simulink model "MCU_Stateflow_Analog"  (R2022b)
settings: Solver=FixedStepDiscrete  StartTime=0.0  StopTime=inf  FixedStep=0.002  RelTol=1e-3
undefined symbols (not defined in the file): ANALOG, cAgeingMode, cCurrentLoopMode, cNoneMode, cParaRecogMode, cSingleBoardMode, cSpeedLoopMode, cTorqueLoopMode, cVvvfOpenMode, FAULT, POWER_ON, STANDBY, TESTBED, VEHICLE, WORKING
libraries: simulink x9, SignalEditorBlockLib x1
(part 3 of 4)

== stateflow chart MCU_Stateflow_Analog/测试/Task_2ms1/Process/McModeManage ==
  (default) -> (junction 10)
  (junction 267) -> (junction 270) [order 1] : [WorkCmdSource_ModeCmd==cTorqueLoopMode]
  (junction 265) -> (junction 267) : [CommandSource == VEHICLE]
  (junction 10) -> (junction 265) [order 2]
  (junction 10) -> (junction 12) [order 1] : [CommandSource == TESTBED]
  (junction 12) -> (junction 40) [order 1] : [WorkCmdSource_ModeCmd==cTorqueLoopMode]
  (junction 270) -> (junction 272) : {WorkStateMc_ModeSelect = cTorqueLoopMode;
      | WorkCmdMc_RunCmd = WorkCmdSource_RunCmd;
      | WorkCmdMc_TorqueCmd = WorkCmdSource_TorqueCmd;}
  (junction 267) -> (junction 274) [order 2] : {WorkStateMc_ModeSelect = cNoneMode;}
  (junction 10) -> (junction 289) [order 3] : [CommandSource == ANALOG]
  (junction 12) -> (junction 47) [order 2]
  (junction 40) -> (junction 43) : {WorkStateMc_ModeSelect = cTorqueLoopMode;
      | WorkCmdMc_RunCmd = WorkCmdSource_RunCmd;
      | WorkCmdMc_TorqueCmd = WorkCmdSource_TorqueCmd;}
  (junction 43) -> (junction 243)
  (junction 243) -> (junction 238)
  (junction 274) -> (junction 272)
  (junction 47) -> (junction 49) [order 1] : [WorkCmdSource_ModeCmd ==cSpeedLoopMode ]
  (junction 272) -> (junction 277) [order 2]
  (junction 272) -> (junction 277) [order 1] : [ZeroTorqueFlag == 1]
      | {WorkStateMc_ModeSelect = cTorqueLoopMode;
      | WorkCmdMc_RunCmd = WorkCmdSource_RunCmd;
      | WorkCmdMc_TorqueCmd = 0;}
  (junction 47) -> (junction 57) [order 2]
  (junction 49) -> (junction 54) : {WorkStateMc_ModeSelect = cSpeedLoopMode;
      | WorkCmdMc_RunCmd = WorkCmdSource_RunCmd;
      | WorkCmdMc_SpeedCmd = WorkCmdSource_SpeedCmd;}
  (junction 328) -> (junction 238) [order 1] : [WorkStateModeSelectBefore ~= cSpeedLoopMode]{SpeedCtrl_SpeedCmdFilter = SpeedCal_speed2ms}
  (junction 289) -> (junction 292)
  (junction 54) -> (junction 328)
  (junction 328) -> (junction 238) [order 2]
  (junction 238) -> (junction 233)
  (junction 292) -> (junction 296) [order 1] : [WorkCmdSource_ModeCmd == cTorqueLoopMode]
  (junction 277) -> (junction 322)
  (junction 292) -> (junction 302) [order 2]
  (junction 296) -> (junction 298) : {WorkStateMc_ModeSelect = cTorqueLoopMode;
      | WorkCmdMc_RunCmd = WorkCmdSource_RunCmd;
      | WorkCmdMc_TorqueCmd = WorkCmdSource_TorqueCmd;}
  (junction 57) -> (junction 59) [order 1] : [WorkCmdSource_ModeCmd ==cCurrentLoopMode ]
  (junction 57) -> (junction 78) [order 2]
  (junction 59) -> (junction 61) : {WorkStateMc_ModeSelect = cCurrentLoopMode;
      | WorkCmdMc_RunCmd = WorkCmdSource_RunCmd;}
  (junction 61) -> (junction 64) [order 1] : [CurrentPolarCoordinatesFlg ==1]
  (junction 298) -> (junction 300)
  (junction 61) -> (junction 71) [order 2] : {WorkCmdMc_IsdCmd = WorkCmdSource_IsdCmd;
      | WorkCmdMc_IsqCmd = WorkCmdSource_IsqCmd}
  (junction 64) -> (junction 66) : {WorkCmdMc_CurrentCmd = WorkCmdSource_CurrentCmd;
      | WorkCmdMc_ThetaCmd = WorkCmdSource_ThetaCmd;}
  (junction 300) -> (junction 308)
  (junction 302) -> (junction 304) [order 1] : [WorkCmdSource_ModeCmd == cSpeedLoopMode]
  (junction 66) -> (junction 71)
  (junction 302) -> (junction 311) [order 2]
  (junction 304) -> (junction 306) : {WorkStateMc_ModeSelect = cSpeedLoopMode;
      | WorkCmdMc_RunCmd = WorkCmdSource_RunCmd;
      | WorkCmdMc_TorqueCmd = WorkCmdSource_SpeedCmd;}
  (junction 71) -> (junction 74)
  (junction 74) -> (junction 233)
  (junction 233) -> (junction 228)
  (junction 306) -> (junction 308)
  (junction 308) -> (junction 313)
  (junction 78) -> (junction 81) [order 1] : [WorkCmdSource_ModeCmd ==cVvvfOpenMode ]
  (junction 78) -> (junction 87) [order 2]
  (junction 81) -> (junction 83) : {WorkStateMc_ModeSelect = cVvvfOpenMode;
      | WorkCmdMc_RunCmd = WorkCmdSource_RunCmd;
      | WorkCmdMc_FreqCmd = WorkCmdSource_FreqCmd;}
  (junction 313) -> (junction 311)
  (junction 311) -> (junction 317) [order 2]
  (junction 311) -> (junction 317) [order 1] : [ZeroTorqueFlag == 1]
      | {WorkStateMc_ModeSelect = cTorqueLoopMode;
      | WorkCmdMc_RunCmd = WorkCmdSource_RunCmd;
      | WorkCmdMc_TorqueCmd = 0;}
  (junction 83) -> (junction 228)
  (junction 228) -> (junction 223)
  (junction 317) -> (junction 319)
  (junction 87) -> (junction 89) [order 1] : [WorkCmdSource_ModeCmd ==cParaRecogMode ]
  (junction 87) -> (junction 94) [order 2]
  (junction 89) -> (junction 91) : {WorkStateMc_ModeSelect = cParaRecogMode;
      | WorkCmdMc_RunCmd = WorkCmdSource_RunCmd;}
  (junction 91) -> (junction 223)
  (junction 223) -> (junction 252)
  (junction 94) -> (junction 96) [order 1] : [WorkCmdSource_ModeCmd ==cSingleBoardMode ]
  (junction 94) -> (junction 100) [order 2]
  (junction 96) -> (junction 98) : {WorkStateMc_ModeSelect = cSingleBoardMode;
      | WorkCmdMc_RunCmd = WorkCmdSource_RunCmd;}
  (junction 98) -> (junction 252)
  (junction 252) -> (junction 254)
  (junction 100) -> (junction 102) [order 1] : [WorkCmdSource_ModeCmd ==cAgeingMode ]
  (junction 100) -> (junction 108) [order 2]
  (junction 102) -> (junction 104) : {WorkStateMc_ModeSelect = cAgeingMode;
      | WorkCmdMc_RunCmd = WorkCmdSource_RunCmd;
      | WorkCmdMc_CurrentCmd = WorkCmdSource_CurrentCmd;
      | WorkCmdMc_ThetaCmd = WorkCmdSource_ThetaCmd;
      | WorkCmdMc_FreqCmd = WorkCmdSource_FreqCmd;}
  (junction 104) -> (junction 254)
  (junction 254) -> (junction 256)
  (junction 108) -> (junction 110) [order 1] : [WorkCmdSource_ModeCmd ==cNoneMode ]
  (junction 108) -> (junction 262) [order 2] : {WorkStateMc_ModeSelect = cNoneMode;}
  (junction 110) -> (junction 112) : {WorkStateMc_ModeSelect = cAgeingMode;
      | WorkCmdMc_RunCmd = WorkCmdSource_RunCmd;}
  (junction 112) -> (junction 256)
  (junction 256) -> (junction 260)
  (junction 260) -> (junction 262)
  (junction 262) -> (junction 259)
  (junction 259) -> (junction 280) [order 2]
  (junction 259) -> (junction 280) [order 1] : [ZeroTorqueFlag == 1]
      | {WorkStateMc_ModeSelect = cTorqueLoopMode;
      | WorkCmdMc_RunCmd = WorkCmdSource_RunCmd;
      | WorkCmdMc_TorqueCmd = 0;}
  (junction 280) -> (junction 324)
  data: WorkCmdSource_ThetaCmd input; CommandSource input; WorkCmdSource_ModeCmd input; WorkCmdSource_RunCmd input; WorkCmdSource_TorqueCmd input; WorkCmdSource_CurrentCmd input; WorkCmdSource_FreqCmd input; WorkCmdSource_IsdCmd input; WorkCmdSource_IsqCmd input; WorkCmdSource_SpeedCmd input; TESTBED parameter; cTorqueLoopMode parameter; WorkStateMc_ModeSelect output =cNoneMode; cSpeedLoopMode parameter; WorkCmdMc_RunCmd output uint16; WorkCmdMc_TorqueCmd output single; WorkCmdMc_SpeedCmd output; cCurrentLoopMode parameter; WorkCmdMc_ThetaCmd output; WorkCmdMc_CurrentCmd output; CurrentPolarCoordinatesFlg input; WorkCmdMc_IsdCmd output; WorkCmdMc_IsqCmd output; cVvvfOpenMode parameter; WorkCmdMc_FreqCmd output; cParaRecogMode parameter; cAgeingMode parameter; cSingleBoardMode parameter; cNoneMode parameter; VEHICLE parameter; ZeroTorqueFlag input; SpeedCal_speed2ms input; ANALOG parameter; WorkStateModeSelectBefore input; SpeedCtrl_SpeedCmdFilter output

== stateflow chart MCU_Stateflow_Analog/测试/Task_2ms1/Process/WorkCmdJudge ==
  (default) -> (junction 1)
  (junction 10) -> (junction 31) [order 1] : [WorkState_TestBedWorkEn == 1]
  (junction 8) -> (junction 10) : [CommandSource ==TESTBED]
  (junction 1) -> (junction 8) [order 2]
  (junction 1) -> (junction 3) [order 1] : [CommandSource==VEHICLE]
  (junction 3) -> (junction 13) [order 1] : [WorkCmdVehicle_RunCmd == 1]
  (junction 31) -> (junction 34) : {WorkCmdSource_RunCmd =WorkCmdTestbed_RunCmd;
      | WorkCmdSource_DischargeCmd = WorkCmdTestbed_DischargeCmd;
      | WorkCmdSource_ModeCmd = WorkCmdTestbed_ModeCmd;
      | WorkCmdSource_TorqueCmd = WorkCmdTestbed_TorqueCmd;
      | WorkCmdSource_SpeedCmd = WorkCmdTestbed_SpeedCmd;
      | WorkCmdSource_CurrentCmd = WorkCmdTestbed_CurrentCmd;
      | WorkCmdSource_ThetaCmd = WorkCmdTestbed_ThetaCmd;
      | WorkCmdSource_IsdCmd = WorkCmdTestbed_IsdCmd;
      | WorkCmdSource_IsqCmd =WorkCmdTestbed_IsqCmd;
      | WorkCmdSource_FreqCmd = WorkCmdTestbed_FreqCmd;}
  (junction 10) -> (junction 36) [order 2] : {WorkCmdSource_RunCmd =0;
      | WorkCmdSource_DischargeCmd = 0;
      | WorkCmdSource_ModeCmd = cNoneMode;
      | WorkCmdSource_TorqueCmd = 0;
      | WorkCmdSource_SpeedCmd = 0;
      | WorkCmdSource_CurrentCmd = 0;
      | WorkCmdSource_ThetaCmd = 0;
      | WorkCmdSource_IsdCmd = 0;
      | WorkCmdSource_IsqCmd =0;
      | WorkCmdSource_FreqCmd = 0;}
  (junction 1) -> (junction 67) [order 3] : [CommandSource == ANALOG]
  (junction 3) -> (junction 28) [order 2] : {WorkCmdSource_RunCmd =0;
      | WorkCmdSource_DischargeCmd = WorkCmdVehicle_DischargeCmd;
      | WorkCmdSource_ModeCmd = cNoneMode;
      | WorkCmdSource_TorqueCmd = 0;
      | WorkCmdSource_SpeedCmd = 0;
      | WorkCmdSource_CurrentCmd = 0;
      | WorkCmdSource_ThetaCmd = 0;
      | WorkCmdSource_IsdCmd = 0;
      | WorkCmdSource_IsqCmd =0;
      | WorkCmdSource_FreqCmd = 0}
  (junction 13) -> (junction 15) : {WorkCmdSource_RunCmd =1;
      | WorkCmdSource_DischargeCmd = WorkCmdVehicle_DischargeCmd;
      | WorkCmdSource_ModeCmd = cTorqueLoopMode;
      | WorkCmdSource_TorqueCmd = WorkCmdVehicle_TorqueCmd
      | WorkCmdSource_SpeedCmd = 0;
      | WorkCmdSource_CurrentCmd = 0;
      | WorkCmdSource_ThetaCmd = 0;
      | WorkCmdSource_IsdCmd = 0;
      | WorkCmdSource_IsqCmd =0;
      | WorkCmdSource_FreqCmd = 0}
  (junction 36) -> (junction 34)
  (junction 28) -> (junction 15)
  (junction 34) -> (junction 56)
  (junction 15) -> (junction 54)
  (junction 67) -> (junction 70) [order 1] : [WorkCmdAnalog_RunCmd == 1]
  (junction 67) -> (junction 80) [order 2] : {WorkCmdSource_RunCmd =0;
      | WorkCmdSource_DischargeCmd = WorkCmdVehicle_DischargeCmd;
      | WorkCmdSource_ModeCmd = cNoneMode;
      | WorkCmdSource_TorqueCmd = 0;
      | WorkCmdSource_SpeedCmd = 0;
      | WorkCmdSource_CurrentCmd = 0;
      | WorkCmdSource_ThetaCmd = 0;
      | WorkCmdSource_IsdCmd = 0;
      | WorkCmdSource_IsqCmd =0;
      | WorkCmdSource_FreqCmd = 0}
  (junction 70) -> (junction 78) : {WorkCmdSource_RunCmd =1;
      | WorkCmdSource_DischargeCmd = 0;
      | WorkCmdSource_ModeCmd = WorkCmdAnalog_ModeCmd;
      | WorkCmdSource_TorqueCmd = WorkCmdAnalog_TorqueCmd;
      | WorkCmdSource_SpeedCmd = WorkCmdAnalog_SpeedCmd;
      | WorkCmdSource_CurrentCmd = 0;
      | WorkCmdSource_ThetaCmd = 0;
      | WorkCmdSource_IsdCmd = 0;
      | WorkCmdSource_IsqCmd =0;
      | WorkCmdSource_FreqCmd = 0}
  (junction 80) -> (junction 78)
  (junction 78) -> (junction 83)
  data: WorkCmdAnalog_ModeCmd input; CommandSource input int16; VEHICLE parameter int16; TESTBED parameter int16; WorkCmdVehicle_RunCmd input uint16; WorkCmdVehicle_DischargeCmd input uint16; WorkCmdSource_DischargeCmd output uint16; WorkCmdSource_RunCmd output uint16; WorkCmdSource_ModeCmd output uint16; cTorqueLoopMode parameter; WorkCmdSource_CurrentCmd output single; WorkCmdSource_FreqCmd output single; WorkCmdSource_IsdCmd output single; WorkCmdSource_IsqCmd output single; WorkCmdSource_SpeedCmd output single; WorkCmdSource_ThetaCmd output single; cNoneMode parameter; WorkState_TestBedWorkEn input uint16; WorkCmdTestbed_RunCmd input uint16; WorkCmdTestbed_DischargeCmd input uint16; WorkCmdTestbed_ModeCmd input uint16; WorkCmdTestbed_SpeedCmd input single; WorkCmdTestbed_CurrentCmd input single; WorkCmdTestbed_FreqCmd input single; WorkCmdTestbed_IsdCmd input single; WorkCmdTestbed_IsqCmd input single; WorkCmdTestbed_ThetaCmd input single; WorkCmdSource_TorqueCmd output single; WorkCmdVehicle_TorqueCmd input single; WorkCmdTestbed_TorqueCmd input single; WorkCmdAnalog_RunCmd input uint16; WorkCmdAnalog_SpeedCmd input; ANALOG parameter; WorkCmdAnalog_TorqueCmd input

== stateflow chart MCU_Stateflow_Analog/测试/Task_2ms1/草稿/Chart ==
  (default) -> (junction 10) : %差一个上一个周期的ModeSelect
      | {}
  (junction 10) -> (junction 12) : [CommandSource == TESTBED]
  (junction 12) -> (junction 40) [order 1] : [WorkCmdSource_ModeCmd==cTorqueLoopMode]
  (junction 12) -> (junction 47) [order 2]
  (junction 40) -> (junction 43) : {WorkStateMc_ModeSelect = cTorqueLoopMode;
      | WorkCmdMc_RunCmd = WorkCmdSource_RunCmd;
      | WorkCmdMc_TorqueCmd = WorkCmdSource_TorqueCmd;}
  (junction 43) -> (junction 243)
  (junction 243) -> (junction 245)
  (junction 47) -> (junction 49) [order 1] : [WorkCmdSource_ModeCmd ==cSpeedLoopMode ]
  (junction 47) -> (junction 57) [order 2]
  (junction 49) -> (junction 54) : {WorkStateMc_ModeSelect = cSpeedLoopMode;
      | WorkCmdMc_RunCmd = WorkCmdSource_RunCmd;
      | WorkCmdMc_SpeedCmd = WorkCmdSource_SpeedCmd;}
  (junction 54) -> (junction 238)
  (junction 238) -> (junction 240)
  (junction 57) -> (junction 59) [order 1] : [WorkCmdSource_ModeCmd ==cCurrentLoopMode ]
  (junction 57) -> (junction 78) [order 2]
  (junction 59) -> (junction 61) : {WorkStateMc_ModeSelect = cCurrentLoopMode;
      | WorkCmdMc_RunCmd = WorkCmdSource_RunCmd;}
  (junction 61) -> (junction 64) [order 1] : [CurrentPolarCoordinatesFlg ==1]
  (junction 61) -> (junction 71) [order 2] : {WorkCmdMc_IsdCmd = WorkCmdSource_IsdCmd;
      | WorkCmdMc_IsqCmd = WorkCmdSource_IsqCmd}
  (junction 64) -> (junction 66) : {WorkCmdMc_CurrentCmd = WorkCmdSource_CurrentCmd;
      | WorkCmdMc_ThetaCmd = WorkCmdSource_ThetaCmd;}
  (junction 66) -> (junction 71)
  (junction 71) -> (junction 74)
  (junction 74) -> (junction 233)
  (junction 233) -> (junction 235)
  (junction 78) -> (junction 81) [order 1] : [WorkCmdSource_ModeCmd ==cVvvfOpenMode ]
  (junction 78) -> (junction 87) [order 2]
  (junction 81) -> (junction 83) : {WorkStateMc_ModeSelect = cVvvfOpenMode;
      | WorkCmdMc_RunCmd = WorkCmdSource_RunCmd;
      | WorkCmdMc_FreqCmd = WorkCmdSource_FreqCmd;}
  (junction 83) -> (junction 228)
  (junction 228) -> (junction 230)
  (junction 87) -> (junction 89) [order 1] : [WorkCmdSource_ModeCmd ==cParaRecogMode ]
  (junction 87) -> (junction 94) [order 2]
  (junction 89) -> (junction 91) : {WorkStateMc_ModeSelect = cParaRecogMode;
      | WorkCmdMc_RunCmd = WorkCmdSource_RunCmd;}
  (junction 91) -> (junction 223)
  (junction 223) -> (junction 225)
  (junction 94) -> (junction 96) [order 1] : [WorkCmdSource_ModeCmd ==cSingleBoardMode ]
  (junction 94) -> (junction 100) [order 2]
  (junction 96) -> (junction 98) : {WorkStateMc_ModeSelect = cSingleBoardMode;
      | WorkCmdMc_RunCmd = WorkCmdSource_RunCmd;}
  (junction 98) -> (junction 218)
  (junction 218) -> (junction 220)
  (junction 100) -> (junction 102) [order 1] : [WorkCmdSource_ModeCmd ==cAgeingMode ]
  (junction 100) -> (junction 108) [order 2]
  (junction 102) -> (junction 104) : {WorkStateMc_ModeSelect = cAgeingMode;
      | WorkCmdMc_RunCmd = WorkCmdSource_RunCmd;
      | WorkCmdMc_CurrentCmd = WorkCmdSource_CurrentCmd;
      | WorkCmdMc_ThetaCmd = WorkCmdSource_ThetaCmd;
      | WorkCmdMc_FreqCmd = WorkCmdSource_FreqCmd;}
  (junction 104) -> (junction 213)
  (junction 213) -> (junction 215)
  (junction 108) -> (junction 110) [order 1] : [WorkCmdSource_ModeCmd ==cNoneMode ]
  (junction 108) -> (junction 114) [order 2] : {WorkStateMc_ModeSelect = cAgeingMode;}
  (junction 110) -> (junction 112) : {WorkStateMc_ModeSelect = cAgeingMode;
      | WorkCmdMc_RunCmd = WorkCmdSource_RunCmd;}
  (junction 112) -> (junction 114)
  (junction 215) -> (junction 112)
  (junction 220) -> (junction 215)
  (junction 225) -> (junction 220)
  (junction 230) -> (junction 225)
  (junction 235) -> (junction 230)
  (junction 240) -> (junction 235)
  (junction 245) -> (junction 240)
  (junction 114) -> (junction 211)
  data: WorkCmdSource_ThetaCmd input; CommandSource input; WorkCmdSource_ModeCmd input; WorkCmdSource_RunCmd input; WorkCmdSource_TorqueCmd input; WorkCmdSource_CurrentCmd input; WorkCmdSource_FreqCmd input; WorkCmdSource_IsdCmd input; WorkCmdSource_IsqCmd input; WorkCmdSource_SpeedCmd input; TESTBED parameter; cTorqueLoopMode parameter; WorkStateMc_ModeSelect output; cSpeedLoopMode parameter; WorkCmdMc_RunCmd output; WorkCmdMc_TorqueCmd output; WorkCmdMc_SpeedCmd output; cCurrentLoopMode parameter; WorkCmdMc_ThetaCmd output; WorkCmdMc_CurrentCmd output; CurrentPolarCoordinatesFlg input; WorkCmdMc_IsdCmd output; WorkCmdMc_IsqCmd output; cVvvfOpenMode parameter; WorkCmdMc_FreqCmd output; cParaRecogMode parameter; cAgeingMode parameter; cSingleBoardMode parameter; cNoneMode parameter

== stateflow chart MCU_Stateflow_Analog/测试/Task_2ms1/草稿/Chart2 ==
  (default) -> (junction 10) : %差一个上一个周期的ModeSelect
  (junction 10) -> (junction 12) [order 1] : [CommandSource == TESTBED]
  (junction 12) -> (junction 40) [order 1] : [WorkCmdSource_ModeCmd==cTorqueLoopMode]
  (junction 10) -> (junction 265) [order 2]
  (junction 12) -> (junction 47) [order 2]
  (junction 40) -> (junction 43) : {WorkStateMc_ModeSelect = cTorqueLoopMode;
      | WorkCmdMc_RunCmd = WorkCmdSource_RunCmd;
      | WorkCmdMc_TorqueCmd = WorkCmdSource_TorqueCmd;}
  (junction 43) -> (junction 243)
  (junction 267) -> (junction 270) [order 1] : [WorkCmdSource_ModeCmd==cTorqueLoopMode]
  (junction 265) -> (junction 267) : [CommandSource == VEHICLE]
  (junction 243) -> (junction 238)
  (junction 270) -> (junction 272) : {WorkStateMc_ModeSelect = cTorqueLoopMode;
      | WorkCmdMc_RunCmd = WorkCmdSource_RunCmd;
      | WorkCmdMc_TorqueCmd = WorkCmdSource_TorqueCmd;}
  (junction 267) -> (junction 274) [order 2] : {WorkStateMc_ModeSelect = cNoneMode;}
  (junction 47) -> (junction 49) [order 1] : [WorkCmdSource_ModeCmd ==cSpeedLoopMode ]
  (junction 47) -> (junction 57) [order 2]
  (junction 49) -> (junction 54) : {WorkStateMc_ModeSelect = cSpeedLoopMode;
      | WorkCmdMc_RunCmd = WorkCmdSource_RunCmd;
      | WorkCmdMc_SpeedCmd = WorkCmdSource_SpeedCmd;}
  (junction 274) -> (junction 272)
  (junction 54) -> (junction 238)
  (junction 272) -> (junction 277)
  (junction 238) -> (junction 233)
  (junction 57) -> (junction 59) [order 1] : [WorkCmdSource_ModeCmd ==cCurrentLoopMode ]
  (junction 57) -> (junction 78) [order 2]
  (junction 59) -> (junction 61) : {WorkStateMc_ModeSelect = cCurrentLoopMode;
      | WorkCmdMc_RunCmd = WorkCmdSource_RunCmd;}
  (junction 61) -> (junction 64) [order 1] : [CurrentPolarCoordinatesFlg ==1]
  (junction 61) -> (junction 71) [order 2] : {WorkCmdMc_IsdCmd = WorkCmdSource_IsdCmd;
      | WorkCmdMc_IsqCmd = WorkCmdSource_IsqCmd}
  (junction 64) -> (junction 66) : {WorkCmdMc_CurrentCmd = WorkCmdSource_CurrentCmd;
      | WorkCmdMc_ThetaCmd = WorkCmdSource_ThetaCmd;}
  (junction 66) -> (junction 71)
  (junction 71) -> (junction 74)
  (junction 74) -> (junction 233)
  (junction 233) -> (junction 228)
  (junction 78) -> (junction 81) [order 1] : [WorkCmdSource_ModeCmd ==cVvvfOpenMode ]
  (junction 78) -> (junction 87) [order 2]
  (junction 81) -> (junction 83) : {WorkStateMc_ModeSelect = cVvvfOpenMode;
      | WorkCmdMc_RunCmd = WorkCmdSource_RunCmd;
      | WorkCmdMc_FreqCmd = WorkCmdSource_FreqCmd;}
  (junction 83) -> (junction 228)
  (junction 228) -> (junction 223)
  (junction 87) -> (junction 89) [order 1] : [WorkCmdSource_ModeCmd ==cParaRecogMode ]
  (junction 87) -> (junction 94) [order 2]
  (junction 89) -> (junction 91) : {WorkStateMc_ModeSelect = cParaRecogMode;
      | WorkCmdMc_RunCmd = WorkCmdSource_RunCmd;}
  (junction 91) -> (junction 223)
  (junction 223) -> (junction 252)
  (junction 94) -> (junction 96) [order 1] : [WorkCmdSource_ModeCmd ==cSingleBoardMode ]
  (junction 94) -> (junction 100) [order 2]
  (junction 96) -> (junction 98) : {WorkStateMc_ModeSelect = cSingleBoardMode;
      | WorkCmdMc_RunCmd = WorkCmdSource_RunCmd;}
  (junction 98) -> (junction 252)
  (junction 252) -> (junction 254)
  (junction 100) -> (junction 102) [order 1] : [WorkCmdSource_ModeCmd ==cAgeingMode ]
  (junction 100) -> (junction 108) [order 2]
  (junction 102) -> (junction 104) : {WorkStateMc_ModeSelect = cAgeingMode;
      | WorkCmdMc_RunCmd = WorkCmdSource_RunCmd;
      | WorkCmdMc_CurrentCmd = WorkCmdSource_CurrentCmd;
      | WorkCmdMc_ThetaCmd = WorkCmdSource_ThetaCmd;
      | WorkCmdMc_FreqCmd = WorkCmdSource_FreqCmd;}
  (junction 104) -> (junction 254)
  (junction 254) -> (junction 256)
  (junction 108) -> (junction 110) [order 1] : [WorkCmdSource_ModeCmd ==cNoneMode ]
  (junction 108) -> (junction 262) [order 2] : {WorkStateMc_ModeSelect = cNoneMode;}
  (junction 110) -> (junction 112) : {WorkStateMc_ModeSelect = cAgeingMode;
      | WorkCmdMc_RunCmd = WorkCmdSource_RunCmd;}
  (junction 112) -> (junction 256)
  (junction 256) -> (junction 260)
  (junction 260) -> (junction 262)
  (junction 262) -> (junction 259)
  data: WorkCmdSource_ThetaCmd input; CommandSource input; WorkCmdSource_ModeCmd input; WorkCmdSource_RunCmd input; WorkCmdSource_TorqueCmd input; WorkCmdSource_CurrentCmd input; WorkCmdSource_FreqCmd input; WorkCmdSource_IsdCmd input; WorkCmdSource_IsqCmd input; WorkCmdSource_SpeedCmd input; TESTBED parameter; cTorqueLoopMode parameter; WorkStateMc_ModeSelect output; cSpeedLoopMode parameter; WorkCmdMc_RunCmd output; WorkCmdMc_TorqueCmd output; WorkCmdMc_SpeedCmd output; cCurrentLoopMode parameter; WorkCmdMc_ThetaCmd output; WorkCmdMc_CurrentCmd output; CurrentPolarCoordinatesFlg input; WorkCmdMc_IsdCmd output; WorkCmdMc_IsqCmd output; cVvvfOpenMode parameter; WorkCmdMc_FreqCmd output; cParaRecogMode parameter; cAgeingMode parameter; cSingleBoardMode parameter; cNoneMode parameter; VEHICLE parameter

== stateflow chart MCU_Stateflow_Analog/测试/Task_2ms1/草稿/MotorState1 ==
  state PowerOn
    WorkState_WorkState = POWER_ON
  state Fault
    WorkState_WorkState = FAULT;
  state StandBy
    WorkState_WorkState = STANDBY;
  state Working
    WorkState_WorkState = WORKING;
  (default) -> PowerOn
  PowerOn -> (junction 21) : [SelfCheck_OverFlg == 1]
  (junction 13) -> Fault : {WorkState_WorkState = FAULT;
      | WorkState_WorkStateBefore = POWER_ON;
      | WorkState_ModeSelect = cNoneMode;}
  (junction 21) -> (junction 13) [order 1] : [ClosePWMFlag == 1]
  (junction 21) -> StandBy [order 2] : {WorkState_WorkState = STANDBY;
      | WorkState_WorkStateBefore = POWER_ON;
      | WorkState_ModeSelect = cNoneMode;}
  (junction 26) -> Fault : {WorkState_WorkState = FAULT;
      | WorkState_WorkStateBefore = STANDBY;
      | WorkState_ModeSelect = cNoneMode}
  StandBy -> (junction 26) [order 1] : [ClosePWMFlag ==1]
  Fault -> (junction 47) : [ClosePWMFlag ==0]
  (junction 47) -> StandBy : {WorkState_WorkState = STANDBY;
      | WorkState_WorkStateBefore = FAULT;
      | WorkState_ModeSelect = cNoneMode}
  StandBy -> (junction 30) [order 2] : [(WorkCmdSource_ModeCmd ~=cNoneMode & WorkCmdSource_RunCmd==true &Precharge_PrechargeOver==true) ||(WormCmdSource_ModeCmd ==cSingleBoardMode)]
  (junction 30) -> Working : {WorkState_WorkState =WORKING;
      | WorkState_WorkStateBefore = STANDBY;}
  (junction 43) -> Fault : {WorkState_WorkState = FAULT;
      | WorkState_WorkStateBefore = WORKING;
      | WorkState_ModeSelect = cNoneMode;}
  Working -> (junction 43) : [ClosePWMFlag==1]
  data: SelfCheck_OverFlg input; POWER_ON parameter; ClosePWMFlag input; FAULT parameter; WorkState_WorkState output; WorkState_WorkStateBefore output; cNoneMode parameter; WorkState_ModeSelect output; STANDBY parameter; cSingleBoardMode parameter; WormCmdSource_ModeCmd input; WorkCmdSource_RunCmd input; WorkCmdSource_ModeCmd input; Precharge_PrechargeOver input; WORKING parameter

== stateflow chart MCU_Stateflow_Analog/测试/Task_2ms1/草稿/MotorState2 ==
  state PowerOn
    WorkState_WorkState = POWER_ON
  state Fault
    WorkState_WorkState = FAULT;
  state StandBy
    WorkState_WorkState = STANDBY;
  state Working
    WorkState_WorkState = WORKING;
  (default) -> PowerOn
  PowerOn -> (junction 21) : [SelfCheck_OverFlg == 1]
  (junction 13) -> Fault : {WorkState_WorkState = FAULT;
      | WorkState_WorkStateBefore = POWER_ON;
      | WorkState_ModeSelect = cNoneMode;}
  (junction 21) -> (junction 13) [order 1] : [ClosePWMFlag == 1]
  (junction 21) -> StandBy [order 2] : {WorkState_WorkState = STANDBY;
      | WorkState_WorkStateBefore = POWER_ON;
      | WorkState_ModeSelect = cNoneMode;}
  (junction 26) -> Fault : {WorkState_WorkState = FAULT;
      | WorkState_WorkStateBefore = STANDBY;
      | WorkState_ModeSelect = cNoneMode}
  StandBy -> (junction 26) [order 1] : [ClosePWMFlag ==1]
  Fault -> (junction 47) : [ClosePWMFlag ==0]
  (junction 47) -> StandBy : {WorkState_WorkState = STANDBY;
      | WorkState_WorkStateBefore = FAULT;
      | WorkState_ModeSelect = cNoneMode}
  StandBy -> (junction 30) [order 2] : [(WorkCmdSource_ModeCmd ~=cNoneMode & WorkCmdSource_RunCmd==true &Precharge_PrechargeOver==true) ||(WormCmdSource_ModeCmd ==cSingleBoardMode)]
  (junction 30) -> Working : {WorkState_WorkState =WORKING;
      | WorkState_WorkStateBefore = STANDBY;}
  (junction 43) -> Fault : {WorkState_WorkState = FAULT;
      | WorkState_WorkStateBefore = WORKING;
      | WorkState_ModeSelect = cNoneMode;}
  Working -> (junction 43) : [ClosePWMFlag==1]
  data: WorkCmdMc_FreqCmd input; WorkCmdMc_IsqCmd input; WorkCmdMc_IsdCmd input; WorkCmdMc_CurrentCmd input; WorkCmdMc_ThetaCmd input; WorkCmdMc_TorqueCmd input; SelfCheck_OverFlg input; POWER_ON parameter; ClosePWMFlag input; FAULT parameter; WorkState_WorkState output; WorkState_WorkStateBefore output; cNoneMode parameter; WorkState_ModeSelect output; STANDBY parameter; cSingleBoardMode parameter; WormCmdSource_ModeCmd input; WorkCmdSource_RunCmd input; WorkCmdSource_ModeCmd input; Precharge_PrechargeOver input; WORKING parameter; WorkStateMc_ModeSelect input; WorkCmdMc_RunCmd input; WorkCmdMc_SpeedCmd input

== stateflow chart MCU_Stateflow_Analog/测试/Task_2ms1/草稿/MotorState3 ==
  state PowerOn
    WorkState_WorkState = POWER_ON
    %WorkCmd_RunCmd = WorkCmdMc_RunCmd;
    %WorkCmd_DischargeCmd = 0;
    %WorkCmd_ModeCmd = cNoneMode;
    %WorkCmd_TorqueCmd = 0;
    %WorkCmd_SpeedCmd = 0;
    %WorkCmd_CurrentCmd = 0;
    %WorkCmd_ThetaCmd = 0;
    %WorkCmd_IsdCmd = 0;
    %WorkCmd_IsqCmd = 0;
    %WorkCmd_FreqCmd = 0;
  state Fault
    %WorkState_WorkState = FAULT;
    %WorkState_WorkState = FAULT;
    %WorkCmd_RunCmd = WorkCmdMc_RunCmd;
    %WorkCmd_DischargeCmd = 0;
    %WorkCmd_ModeCmd = cNoneMode;
    %WorkCmd_TorqueCmd = 0;
    %WorkCmd_SpeedCmd = 0;
    %WorkCmd_CurrentCmd = 0;
    %WorkCmd_ThetaCmd = 0;
    %WorkCmd_IsdCmd = 0;
    %WorkCmd_IsqCmd = 0;
    %WorkCmd_FreqCmd = 0;
  state StandBy
    WorkState_WorkState = STANDBY;
  state Working
    WorkState_WorkState = WORKING;
  (default) -> PowerOn
  PowerOn -> (junction 21) : [SelfCheck_OverFlg == 1]
  (junction 13) -> Fault : {WorkState_WorkState = FAULT;
      | WorkState_WorkStateBefore = POWER_ON;
      | WorkState_ModeSelect = cNoneMode;}
  (junction 21) -> (junction 13) [order 1] : [ClosePWMFlag == 1]
  (junction 21) -> StandBy [order 2] : {WorkState_WorkState = STANDBY;
      | WorkState_WorkStateBefore = POWER_ON;
      | WorkState_ModeSelect = cNoneMode;}
  StandBy -> (junction 26) [order 1] : [ClosePWMFlag ==1]
  (junction 26) -> Fault : {WorkState_WorkState = FAULT;
      | WorkState_WorkStateBefore = STANDBY;
      | WorkState_ModeSelect = cNoneMode}
  Fault -> (junction 47) : [ClosePWMFlag ==0]
  (junction 47) -> StandBy : {WorkState_WorkState = STANDBY;
      | WorkState_WorkStateBefore = FAULT;
      | WorkState_ModeSelect = cNoneMode}
  StandBy -> (junction 30) [order 2] : [(WorkCmdSource_ModeCmd ~=cNoneMode & WorkCmdSource_RunCmd==true &Precharge_PrechargeOver==true) ||(WorkCmdSource_ModeCmd ==cSingleBoardMode)]
  (junction 72) -> StandBy : {WorkState_WorkState = STANDBY;
      | WorkState_WorkStateBefore = WORKING;
      | WorkState_ModeSelect = cNoneMode;}
  (junction 30) -> Working : {WorkState_WorkState =WORKING;
      | WorkState_WorkStateBefore = STANDBY;}
  Working -> (junction 72) [order 2] : [(WorkCmdSource_RunCmd ==false & WorkState_ModeSelect ~= cSingleBoardMode) || (WorkState_ModeSelect == cNoneMode)]
  (junction 43) -> Fault : {WorkState_WorkState = FAULT;
      | WorkState_WorkStateBefore = WORKING;
      | WorkState_ModeSelect = cNoneMode;}
  Working -> (junction 43) [order 1] : [ClosePWMFlag==1]
  data: SelfCheck_OverFlg input; POWER_ON parameter; ClosePWMFlag input; FAULT parameter; WorkState_WorkState output; WorkState_WorkStateBefore output; cNoneMode parameter; WorkState_ModeSelect output; STANDBY parameter; cSingleBoardMode parameter; WorkCmdSource_RunCmd input; WorkCmdSource_ModeCmd input; Precharge_PrechargeOver input; WORKING parameter

== stateflow chart MCU_Stateflow_Analog/测试/Task_2ms1/草稿/MotorState4 ==
  state PowerOn
    %包括Sensor_Self_Check和Ctrl_Reset
    WorkState_WorkState = POWER_ON
  state Fault
    %WorkState_WorkState = FAULT;
    %{
    WorkState_WorkState = FAULT;
    WorkCmd_RunCmd = WorkCmdMc_RunCmd;
    WorkCmd_DischargeCmd = 0;
    WorkCmd_ModeCmd = cNoneMode;
    WorkCmd_TorqueCmd = 0;
    WorkCmd_SpeedCmd = 0;
    WorkCmd_CurrentCmd = 0;
    WorkCmd_ThetaCmd = 0;
    WorkCmd_IsdCmd = 0;
    WorkCmd_IsqCmd = 0;
    WorkCmd_FreqCmd = 0;
    %}
  state StandBy
    WorkState_WorkState = STANDBY;
  state Working
    WorkState_WorkState = WORKING;
  (default) -> PowerOn
  PowerOn -> (junction 21) : [SelfCheck_OverFlg == 1]
  (junction 13) -> Fault : {WorkState_WorkState = FAULT;
      | WorkState_WorkStateBefore = POWER_ON;
      | WorkState_ModeSelect = cNoneMode;}
  (junction 21) -> (junction 13) [order 1] : [ClosePWMFlag == 1]
  (junction 21) -> StandBy [order 2] : {
      | WorkState_WorkState = STANDBY;
      | WorkState_WorkStateBefore = POWER_ON;
      | WorkState_ModeSelect = cNoneMode;}
  StandBy -> (junction 26) [order 1] : [ClosePWMFlag ==1]
  (junction 26) -> Fault : {WorkState_WorkState = FAULT;
      | WorkState_WorkStateBefore = STANDBY;
      | WorkState_ModeSelect = cNoneMode}
  Fault -> (junction 47) : [ClosePWMFlag ==0]
  (junction 47) -> StandBy : {WorkState_WorkState = STANDBY;
      | WorkState_WorkStateBefore = FAULT;
      | WorkState_ModeSelect = cNoneMode}
  StandBy -> (junction 30) [order 2] : [(WorkCmdSource_ModeCmd ~=cNoneMode & WorkCmdSource_RunCmd==true &Precharge_PrechargeOver==true) ||(WorkCmdSource_ModeCmd ==cSingleBoardMode)]
  (junction 72) -> StandBy : {WorkState_WorkState = STANDBY;
      | WorkState_WorkStateBefore = POWER_ON;
      | WorkState_ModeSelect = cNoneMode;}
  (junction 30) -> Working : {WorkState_WorkState =WORKING;
      | WorkState_WorkStateBefore = STANDBY;}
  Working -> (junction 72) [order 2] : [(WorkCmdSource_RunCmd ==false & WorkState_ModeSelect ~= cSingleBoardMode) || (WorkState_ModeSelect == cNoneMode)]
  (junction 43) -> Fault : {WorkState_WorkState = FAULT;
      | WorkState_WorkStateBefore = WORKING;
      | WorkState_ModeSelect = cNoneMode;}
  Working -> (junction 43) [order 1] : [ClosePWMFlag==1]
  data: SelfCheck_OverFlg input; POWER_ON parameter; ClosePWMFlag input; FAULT parameter; WorkState_WorkState output; WorkState_WorkStateBefore output; cNoneMode parameter; WorkState_ModeSelect output; STANDBY parameter; cSingleBoardMode parameter; WorkCmdSource_RunCmd input; WorkCmdSource_ModeCmd input; Precharge_PrechargeOver input; WORKING parameter

== stateflow chart MCU_Stateflow_Analog/测试/Task_2ms2/MotorState ==
  state PowerOn
    %包括Sensor_Self_Check和Ctrl_Reset
    WorkState_WorkState = POWER_ON;
  state Fault
    %WorkState_WorkState = FAULT;
    %{
    WorkState_WorkState = FAULT;
    WorkCmd_RunCmd = WorkCmdMc_RunCmd;
    WorkCmd_DischargeCmd = 0;
    WorkCmd_ModeCmd = cNoneMode;
    WorkCmd_TorqueCmd = 0;
    WorkCmd_SpeedCmd = 0;
    WorkCmd_CurrentCmd = 0;
    WorkCmd_ThetaCmd = 0;
    WorkCmd_IsdCmd = 0;
    WorkCmd_IsqCmd = 0;
    WorkCmd_FreqCmd = 0;
    %}
  state StandBy
    WorkState_WorkState = STANDBY;
  state Working
    WorkState_WorkState = WORKING;
  (default) -> PowerOn
  PowerOn -> (junction 21) : [SelfCheck_OverFlg == 1]
  (junction 13) -> Fault : {
      | WorkState_WorkState = FAULT;
      | WorkState_WorkStateBefore = POWER_ON;
      | %WorkState_ModeSelect = cNoneMode;
      | }
  (junction 21) -> (junction 13) [order 1] : [ClosePWMFlag == 1]
  (junction 21) -> StandBy [order 2] : {
      | WorkState_WorkState = STANDBY;
      | WorkState_WorkStateBefore = POWER_ON;
      | %WorkState_ModeSelect = cNoneMode;
      | }
  StandBy -> (junction 26) [order 1] : [ClosePWMFlag ==1]
  (junction 26) -> Fault : {
      | WorkState_WorkState = FAULT;
      | WorkState_WorkStateBefore = STANDBY;
      | %WorkState_ModeSelect = cNoneMode
      | }
  Fault -> (junction 47) : [ClosePWMFlag ==0]
  (junction 47) -> StandBy : {
      | WorkState_WorkState = STANDBY;
      | WorkState_WorkStateBefore = FAULT;
      | %WorkState_ModeSelect = cNoneMode
      | }
  StandBy -> (junction 30) [order 2] : [(WorkCmdSource_ModeCmd ~=cNoneMode & WorkCmdSource_RunCmd==true &Precharge_PrechargeOver==true) ||(WorkCmdSource_ModeCmd ==cSingleBoardMode)]
  (junction 72) -> StandBy : {
      | WorkState_WorkState = STANDBY;
      | WorkState_WorkStateBefore = POWER_ON;
      | %WorkState_ModeSelect = cNoneMode;
      | }
  (junction 30) -> Working : {WorkState_WorkState =WORKING;
      | WorkState_WorkStateBefore = STANDBY;}
  Working -> (junction 72) [order 2] : %[(WorkCmdSource_RunCmd ==false & WorkState_ModeSelect ~= cSingleBoardMode) || (WorkState_ModeSelect == cNoneMode)]
      | [(WorkCmdSource_RunCmd ==false & WorkStateMc_ModeSelect ~= cSingleBoardMode) || (WorkStateMc_ModeSelect == cNoneMode)]
  (junction 43) -> Fault : {WorkState_WorkState = FAULT;
      | WorkState_WorkStateBefore = WORKING;
      | %WorkState_ModeSelect = cNoneMode;
      | }
  Working -> (junction 43) [order 1] : [ClosePWMFlag==1]
  data: SelfCheck_OverFlg input; POWER_ON parameter; ClosePWMFlag input; FAULT parameter; WorkState_WorkState output; WorkState_WorkStateBefore output; cNoneMode parameter; STANDBY parameter; cSingleBoardMode parameter; WorkCmdSource_RunCmd input; WorkCmdSource_ModeCmd input; Precharge_PrechargeOver input; WORKING parameter; WorkStateMc_ModeSelect input

== stateflow chart MCU_Stateflow_Analog/测试/Task_2ms2/Process/McModeManage ==
  (default) -> (junction 10)
  (junction 267) -> (junction 270) [order 1] : [WorkCmdSource_ModeCmd==cTorqueLoopMode]
  (junction 265) -> (junction 267) : [CommandSource == VEHICLE]
  (junction 10) -> (junction 265) [order 2]
  (junction 10) -> (junction 12) [order 1] : [CommandSource == TESTBED]
  (junction 12) -> (junction 40) [order 1] : [WorkCmdSource_ModeCmd==cTorqueLoopMode]
  (junction 270) -> (junction 272) : {WorkStateMc_ModeSelect = cTorqueLoopMode;
      | WorkCmdMc_RunCmd = WorkCmdSource_RunCmd;
      | WorkCmdMc_TorqueCmd = WorkCmdSource_TorqueCmd;}
  (junction 267) -> (junction 274) [order 2] : {WorkStateMc_ModeSelect = cNoneMode;}
  (junction 10) -> (junction 289) [order 3] : [CommandSource == ANALOG]
  (junction 12) -> (junction 47) [order 2]
  (junction 40) -> (junction 43) : {WorkStateMc_ModeSelect = cTorqueLoopMode;
      | WorkCmdMc_RunCmd = WorkCmdSource_RunCmd;
      | WorkCmdMc_TorqueCmd = WorkCmdSource_TorqueCmd;}
  (junction 43) -> (junction 243)
  (junction 243) -> (junction 238)
  (junction 274) -> (junction 272)
  (junction 47) -> (junction 49) [order 1] : [WorkCmdSource_ModeCmd ==cSpeedLoopMode ]
  (junction 272) -> (junction 277) [order 2]
  (junction 272) -> (junction 277) [order 1] : [ZeroTorqueFlag == 1]
      | {WorkStateMc_ModeSelect = cTorqueLoopMode;
      | WorkCmdMc_RunCmd = WorkCmdSource_RunCmd;
      | WorkCmdMc_TorqueCmd = 0;}
  (junction 47) -> (junction 57) [order 2]
  (junction 49) -> (junction 54) : {WorkStateMc_ModeSelect = cSpeedLoopMode;
      | WorkCmdMc_RunCmd = WorkCmdSource_RunCmd;
      | WorkCmdMc_SpeedCmd = WorkCmdSource_SpeedCmd;}
  (junction 328) -> (junction 238) [order 1] : [WorkStateModeSelectBefore ~= cSpeedLoopMode]{SpeedCtrl_SpeedCmdFilter = SpeedCal_speed2ms}
  (junction 289) -> (junction 292)
  (junction 54) -> (junction 328)
  (junction 328) -> (junction 238) [order 2]
  (junction 238) -> (junction 233)
  (junction 292) -> (junction 296) [order 1] : [WorkCmdSource_ModeCmd == cTorqueLoopMode]
  (junction 277) -> (junction 322)
  (junction 292) -> (junction 302) [order 2]
  (junction 296) -> (junction 298) : {WorkStateMc_ModeSelect = cTorqueLoopMode;
      | WorkCmdMc_RunCmd = WorkCmdSource_RunCmd;
      | WorkCmdMc_TorqueCmd = WorkCmdSource_TorqueCmd;}
  (junction 57) -> (junction 59) [order 1] : [WorkCmdSource_ModeCmd ==cCurrentLoopMode ]
  (junction 57) -> (junction 78) [order 2]
  (junction 59) -> (junction 61) : {WorkStateMc_ModeSelect = cCurrentLoopMode;
      | WorkCmdMc_RunCmd = WorkCmdSource_RunCmd;}
  (junction 61) -> (junction 64) [order 1] : [CurrentPolarCoordinatesFlg ==1]
  (junction 298) -> (junction 300)
  (junction 61) -> (junction 71) [order 2] : {WorkCmdMc_IsdCmd = WorkCmdSource_IsdCmd;
      | WorkCmdMc_IsqCmd = WorkCmdSource_IsqCmd}
  (junction 64) -> (junction 66) : {WorkCmdMc_CurrentCmd = WorkCmdSource_CurrentCmd;
      | WorkCmdMc_ThetaCmd = WorkCmdSource_ThetaCmd;}
  (junction 300) -> (junction 308)
  (junction 302) -> (junction 304) [order 1] : [WorkCmdSource_ModeCmd == cSpeedLoopMode]
  (junction 66) -> (junction 71)
  (junction 302) -> (junction 311) [order 2]
  (junction 304) -> (junction 306) : {WorkStateMc_ModeSelect = cSpeedLoopMode;
      | WorkCmdMc_RunCmd = WorkCmdSource_RunCmd;
      | WorkCmdMc_TorqueCmd = WorkCmdSource_SpeedCmd;}
  (junction 71) -> (junction 74)
  (junction 74) -> (junction 233)
  (junction 233) -> (junction 228)
  (junction 306) -> (junction 308)
  (junction 308) -> (junction 313)
  (junction 78) -> (junction 81) [order 1] : [WorkCmdSource_ModeCmd ==cVvvfOpenMode ]
  (junction 78) -> (junction 87) [order 2]
  (junction 81) -> (junction 83) : {WorkStateMc_ModeSelect = cVvvfOpenMode;
      | WorkCmdMc_RunCmd = WorkCmdSource_RunCmd;
      | WorkCmdMc_FreqCmd = WorkCmdSource_FreqCmd;}
  (junction 313) -> (junction 311)
  (junction 311) -> (junction 317) [order 2]
  (junction 311) -> (junction 317) [order 1] : [ZeroTorqueFlag == 1]
      | {WorkStateMc_ModeSelect = cTorqueLoopMode;
      | WorkCmdMc_RunCmd = WorkCmdSource_RunCmd;
      | WorkCmdMc_TorqueCmd = 0;}
  (junction 83) -> (junction 228)
  (junction 228) -> (junction 223)
  (junction 317) -> (junction 319)
  (junction 87) -> (junction 89) [order 1] : [WorkCmdSource_ModeCmd ==cParaRecogMode ]
  (junction 87) -> (junction 94) [order 2]
  (junction 89) -> (junction 91) : {WorkStateMc_ModeSelect = cParaRecogMode;
      | WorkCmdMc_RunCmd = WorkCmdSource_RunCmd;}
  (junction 91) -> (junction 223)
  (junction 223) -> (junction 252)
  (junction 94) -> (junction 96) [order 1] : [WorkCmdSource_ModeCmd ==cSingleBoardMode ]
  (junction 94) -> (junction 100) [order 2]
  (junction 96) -> (junction 98) : {WorkStateMc_ModeSelect = cSingleBoardMode;
      | WorkCmdMc_RunCmd = WorkCmdSource_RunCmd;}
  (junction 98) -> (junction 252)
  (junction 252) -> (junction 254)
  (junction 100) -> (junction 102) [order 1] : [WorkCmdSource_ModeCmd ==cAgeingMode ]
  (junction 100) -> (junction 108) [order 2]
  (junction 102) -> (junction 104) : {WorkStateMc_ModeSelect = cAgeingMode;
      | WorkCmdMc_RunCmd = WorkCmdSource_RunCmd;
      | WorkCmdMc_CurrentCmd = WorkCmdSource_CurrentCmd;
      | WorkCmdMc_ThetaCmd = WorkCmdSource_ThetaCmd;
      | WorkCmdMc_FreqCmd = WorkCmdSource_FreqCmd;}
  (junction 104) -> (junction 254)
  (junction 254) -> (junction 256)
  (junction 108) -> (junction 110) [order 1] : [WorkCmdSource_ModeCmd ==cNoneMode ]
  (junction 108) -> (junction 262) [order 2] : {WorkStateMc_ModeSelect = cNoneMode;}
  (junction 110) -> (junction 112) : {WorkStateMc_ModeSelect = cAgeingMode;
      | WorkCmdMc_RunCmd = WorkCmdSource_RunCmd;}
  (junction 112) -> (junction 256)
  (junction 256) -> (junction 260)
  (junction 260) -> (junction 262)
  (junction 262) -> (junction 259)
  (junction 259) -> (junction 280) [order 2]
  (junction 259) -> (junction 280) [order 1] : [ZeroTorqueFlag == 1]
      | {WorkStateMc_ModeSelect = cTorqueLoopMode;
      | WorkCmdMc_RunCmd = WorkCmdSource_RunCmd;
      | WorkCmdMc_TorqueCmd = 0;}
  (junction 280) -> (junction 324)
  data: WorkCmdSource_ThetaCmd input; CommandSource input; WorkCmdSource_ModeCmd input; WorkCmdSource_RunCmd input; WorkCmdSource_TorqueCmd input; WorkCmdSource_CurrentCmd input; WorkCmdSource_FreqCmd input; WorkCmdSource_IsdCmd input; WorkCmdSource_IsqCmd input; WorkCmdSource_SpeedCmd input; TESTBED parameter; cTorqueLoopMode parameter; WorkStateMc_ModeSelect output =cNoneMode; cSpeedLoopMode parameter; WorkCmdMc_RunCmd output uint16; WorkCmdMc_TorqueCmd output single; WorkCmdMc_SpeedCmd output; cCurrentLoopMode parameter; WorkCmdMc_ThetaCmd output; WorkCmdMc_CurrentCmd output; CurrentPolarCoordinatesFlg input; WorkCmdMc_IsdCmd output; WorkCmdMc_IsqCmd output; cVvvfOpenMode parameter; WorkCmdMc_FreqCmd output; cParaRecogMode parameter; cAgeingMode parameter; cSingleBoardMode parameter; cNoneMode parameter; VEHICLE parameter; ZeroTorqueFlag input; SpeedCal_speed2ms input; ANALOG parameter; WorkStateModeSelectBefore input; SpeedCtrl_SpeedCmdFilter output

== stateflow chart MCU_Stateflow_Analog/测试/Task_2ms2/Process/WorkCmdJudge ==
  (default) -> (junction 1)
  (junction 10) -> (junction 31) [order 1] : [WorkState_TestBedWorkEn == 1]
  (junction 8) -> (junction 10) : [CommandSource ==TESTBED]
  (junction 1) -> (junction 8) [order 2]
  (junction 1) -> (junction 3) [order 1] : [CommandSource==VEHICLE]
  (junction 3) -> (junction 13) [order 1] : [WorkCmdVehicle_RunCmd == 1]
  (junction 31) -> (junction 34) : {WorkCmdSource_RunCmd =WorkCmdTestbed_RunCmd;
      | WorkCmdSource_DischargeCmd = WorkCmdTestbed_DischargeCmd;
      | WorkCmdSource_ModeCmd = WorkCmdTestbed_ModeCmd;
      | WorkCmdSource_TorqueCmd = WorkCmdTestbed_TorqueCmd;
      | WorkCmdSource_SpeedCmd = WorkCmdTestbed_SpeedCmd;
      | WorkCmdSource_CurrentCmd = WorkCmdTestbed_CurrentCmd;
      | WorkCmdSource_ThetaCmd = WorkCmdTestbed_ThetaCmd;
      | WorkCmdSource_IsdCmd = WorkCmdTestbed_IsdCmd;
      | WorkCmdSource_IsqCmd =WorkCmdTestbed_IsqCmd;
      | WorkCmdSource_FreqCmd = WorkCmdTestbed_FreqCmd;}
  (junction 10) -> (junction 36) [order 2] : {WorkCmdSource_RunCmd =0;
      | WorkCmdSource_DischargeCmd = 0;
      | WorkCmdSource_ModeCmd = cNoneMode;
      | WorkCmdSource_TorqueCmd = 0;
      | WorkCmdSource_SpeedCmd = 0;
      | WorkCmdSource_CurrentCmd = 0;
      | WorkCmdSource_ThetaCmd = 0;
      | WorkCmdSource_IsdCmd = 0;
      | WorkCmdSource_IsqCmd =0;
      | WorkCmdSource_FreqCmd = 0;}
  (junction 1) -> (junction 67) [order 3] : [CommandSource == ANALOG]
  (junction 3) -> (junction 28) [order 2] : {WorkCmdSource_RunCmd =0;
      | WorkCmdSource_DischargeCmd = WorkCmdVehicle_DischargeCmd;
      | WorkCmdSource_ModeCmd = cNoneMode;
      | WorkCmdSource_TorqueCmd = 0;
      | WorkCmdSource_SpeedCmd = 0;
      | WorkCmdSource_CurrentCmd = 0;
      | WorkCmdSource_ThetaCmd = 0;
      | WorkCmdSource_IsdCmd = 0;
      | WorkCmdSource_IsqCmd =0;
      | WorkCmdSource_FreqCmd = 0}
  (junction 13) -> (junction 15) : {WorkCmdSource_RunCmd =1;
      | WorkCmdSource_DischargeCmd = WorkCmdVehicle_DischargeCmd;
      | WorkCmdSource_ModeCmd = cTorqueLoopMode;
      | WorkCmdSource_TorqueCmd = WorkCmdVehicle_TorqueCmd
      | WorkCmdSource_SpeedCmd = 0;
      | WorkCmdSource_CurrentCmd = 0;
      | WorkCmdSource_ThetaCmd = 0;
      | WorkCmdSource_IsdCmd = 0;
      | WorkCmdSource_IsqCmd =0;
      | WorkCmdSource_FreqCmd = 0}
  (junction 36) -> (junction 34)
  (junction 28) -> (junction 15)
  (junction 34) -> (junction 56)
  (junction 15) -> (junction 54)
  (junction 67) -> (junction 70) [order 1] : [WorkCmdAnalog_RunCmd == 1]
  (junction 67) -> (junction 80) [order 2] : {WorkCmdSource_RunCmd =0;
      | WorkCmdSource_DischargeCmd = WorkCmdVehicle_DischargeCmd;
      | WorkCmdSource_ModeCmd = cNoneMode;
      | WorkCmdSource_TorqueCmd = 0;
      | WorkCmdSource_SpeedCmd = 0;
      | WorkCmdSource_CurrentCmd = 0;
      | WorkCmdSource_ThetaCmd = 0;
      | WorkCmdSource_IsdCmd = 0;
      | WorkCmdSource_IsqCmd =0;
      | WorkCmdSource_FreqCmd = 0}
  (junction 70) -> (junction 78) : {WorkCmdSource_RunCmd =1;
      | WorkCmdSource_DischargeCmd = 0;
      | WorkCmdSource_ModeCmd = WorkCmdAnalog_ModeCmd;
      | WorkCmdSource_TorqueCmd = WorkCmdAnalog_TorqueCmd;
      | WorkCmdSource_SpeedCmd = WorkCmdAnalog_SpeedCmd;
      | WorkCmdSource_CurrentCmd = 0;
      | WorkCmdSource_ThetaCmd = 0;
      | WorkCmdSource_IsdCmd = 0;
      | WorkCmdSource_IsqCmd =0;
      | WorkCmdSource_FreqCmd = 0}
  (junction 80) -> (junction 78)
  (junction 78) -> (junction 83)
  data: WorkCmdAnalog_ModeCmd input; CommandSource input int16; VEHICLE parameter int16; TESTBED parameter int16; WorkCmdVehicle_RunCmd input uint16; WorkCmdVehicle_DischargeCmd input uint16; WorkCmdSource_DischargeCmd output uint16; WorkCmdSource_RunCmd output uint16; WorkCmdSource_ModeCmd output uint16; cTorqueLoopMode parameter; WorkCmdSource_CurrentCmd output single; WorkCmdSource_FreqCmd output single; WorkCmdSource_IsdCmd output single; WorkCmdSource_IsqCmd output single; WorkCmdSource_SpeedCmd output single; WorkCmdSource_ThetaCmd output single; cNoneMode parameter; WorkState_TestBedWorkEn input uint16; WorkCmdTestbed_RunCmd input uint16; WorkCmdTestbed_DischargeCmd input uint16; WorkCmdTestbed_ModeCmd input uint16; WorkCmdTestbed_SpeedCmd input single; WorkCmdTestbed_CurrentCmd input single; WorkCmdTestbed_FreqCmd input single; WorkCmdTestbed_IsdCmd input single; WorkCmdTestbed_IsqCmd input single; WorkCmdTestbed_ThetaCmd input single; WorkCmdSource_TorqueCmd output single; WorkCmdVehicle_TorqueCmd input single; WorkCmdTestbed_TorqueCmd input single; WorkCmdAnalog_RunCmd input uint16; WorkCmdAnalog_SpeedCmd input; ANALOG parameter; WorkCmdAnalog_TorqueCmd input

== stateflow chart MCU_Stateflow_Analog/测试/Task_2ms2/草稿/Chart ==
  (default) -> (junction 10) : %差一个上一个周期的ModeSelect
      | {}
  (junction 10) -> (junction 12) : [CommandSource == TESTBED]
  (junction 12) -> (junction 40) [order 1] : [WorkCmdSource_ModeCmd==cTorqueLoopMode]
  (junction 12) -> (junction 47) [order 2]
  (junction 40) -> (junction 43) : {WorkStateMc_ModeSelect = cTorqueLoopMode;
      | WorkCmdMc_RunCmd = WorkCmdSource_RunCmd;
      | WorkCmdMc_TorqueCmd = WorkCmdSource_TorqueCmd;}
  (junction 43) -> (junction 243)
  (junction 243) -> (junction 245)
  (junction 47) -> (junction 49) [order 1] : [WorkCmdSource_ModeCmd ==cSpeedLoopMode ]
  (junction 47) -> (junction 57) [order 2]
  (junction 49) -> (junction 54) : {WorkStateMc_ModeSelect = cSpeedLoopMode;
      | WorkCmdMc_RunCmd = WorkCmdSource_RunCmd;
      | WorkCmdMc_SpeedCmd = WorkCmdSource_SpeedCmd;}
  (junction 54) -> (junction 238)
  (junction 238) -> (junction 240)
  (junction 57) -> (junction 59) [order 1] : [WorkCmdSource_ModeCmd ==cCurrentLoopMode ]
  (junction 57) -> (junction 78) [order 2]
  (junction 59) -> (junction 61) : {WorkStateMc_ModeSelect = cCurrentLoopMode;
      | WorkCmdMc_RunCmd = WorkCmdSource_RunCmd;}
  (junction 61) -> (junction 64) [order 1] : [CurrentPolarCoordinatesFlg ==1]
  (junction 61) -> (junction 71) [order 2] : {WorkCmdMc_IsdCmd = WorkCmdSource_IsdCmd;
      | WorkCmdMc_IsqCmd = WorkCmdSource_IsqCmd}
  (junction 64) -> (junction 66) : {WorkCmdMc_CurrentCmd = WorkCmdSource_CurrentCmd;
      | WorkCmdMc_ThetaCmd = WorkCmdSource_ThetaCmd;}
  (junction 66) -> (junction 71)
  (junction 71) -> (junction 74)
  (junction 74) -> (junction 233)
  (junction 233) -> (junction 235)
  (junction 78) -> (junction 81) [order 1] : [WorkCmdSource_ModeCmd ==cVvvfOpenMode ]
  (junction 78) -> (junction 87) [order 2]
  (junction 81) -> (junction 83) : {WorkStateMc_ModeSelect = cVvvfOpenMode;
      | WorkCmdMc_RunCmd = WorkCmdSource_RunCmd;
      | WorkCmdMc_FreqCmd = WorkCmdSource_FreqCmd;}
  (junction 83) -> (junction 228)
  (junction 228) -> (junction 230)
  (junction 87) -> (junction 89) [order 1] : [WorkCmdSource_ModeCmd ==cParaRecogMode ]
  (junction 87) -> (junction 94) [order 2]
  (junction 89) -> (junction 91) : {WorkStateMc_ModeSelect = cParaRecogMode;
      | WorkCmdMc_RunCmd = WorkCmdSource_RunCmd;}
  (junction 91) -> (junction 223)
  (junction 223) -> (junction 225)
  (junction 94) -> (junction 96) [order 1] : [WorkCmdSource_ModeCmd ==cSingleBoardMode ]
  (junction 94) -> (junction 100) [order 2]
  (junction 96) -> (junction 98) : {WorkStateMc_ModeSelect = cSingleBoardMode;
      | WorkCmdMc_RunCmd = WorkCmdSource_RunCmd;}
  (junction 98) -> (junction 218)
  (junction 218) -> (junction 220)
  (junction 100) -> (junction 102) [order 1] : [WorkCmdSource_ModeCmd ==cAgeingMode ]
  (junction 100) -> (junction 108) [order 2]
  (junction 102) -> (junction 104) : {WorkStateMc_ModeSelect = cAgeingMode;
      | WorkCmdMc_RunCmd = WorkCmdSource_RunCmd;
      | WorkCmdMc_CurrentCmd = WorkCmdSource_CurrentCmd;
      | WorkCmdMc_ThetaCmd = WorkCmdSource_ThetaCmd;
      | WorkCmdMc_FreqCmd = WorkCmdSource_FreqCmd;}
  (junction 104) -> (junction 213)
  (junction 213) -> (junction 215)
  (junction 108) -> (junction 110) [order 1] : [WorkCmdSource_ModeCmd ==cNoneMode ]
  (junction 108) -> (junction 114) [order 2] : {WorkStateMc_ModeSelect = cAgeingMode;}
  (junction 110) -> (junction 112) : {WorkStateMc_ModeSelect = cAgeingMode;
      | WorkCmdMc_RunCmd = WorkCmdSource_RunCmd;}
  (junction 112) -> (junction 114)
  (junction 215) -> (junction 112)
  (junction 220) -> (junction 215)
  (junction 225) -> (junction 220)
  (junction 230) -> (junction 225)
  (junction 235) -> (junction 230)
  (junction 240) -> (junction 235)
  (junction 245) -> (junction 240)
  (junction 114) -> (junction 211)
  data: WorkCmdSource_ThetaCmd input; CommandSource input; WorkCmdSource_ModeCmd input; WorkCmdSource_RunCmd input; WorkCmdSource_TorqueCmd input; WorkCmdSource_CurrentCmd input; WorkCmdSource_FreqCmd input; WorkCmdSource_IsdCmd input; WorkCmdSource_IsqCmd input; WorkCmdSource_SpeedCmd input; TESTBED parameter; cTorqueLoopMode parameter; WorkStateMc_ModeSelect output; cSpeedLoopMode parameter; WorkCmdMc_RunCmd output; WorkCmdMc_TorqueCmd output; WorkCmdMc_SpeedCmd output; cCurrentLoopMode parameter; WorkCmdMc_ThetaCmd output; WorkCmdMc_CurrentCmd output; CurrentPolarCoordinatesFlg input; WorkCmdMc_IsdCmd output; WorkCmdMc_IsqCmd output; cVvvfOpenMode parameter; WorkCmdMc_FreqCmd output; cParaRecogMode parameter; cAgeingMode parameter; cSingleBoardMode parameter; cNoneMode parameter
